simulink model "HW01_Tirel_Sim"  (R2020b)
settings: Solver=VariableStepAuto  StartTime=0.0  StopTime=1  RelTol=1e-3
values from neighbouring files (symbols this model uses):
  Bm = 1.02*10^-9    (= 1.02e-09)    [HW01_Tirel_Mat.m]
  Jm = 9.5*10^-10    (= 9.5e-10)    [HW01_Tirel_Mat.m]
  ke = 0.000114    [HW01_Tirel_Mat.m]
  km = 0.00109    [HW01_Tirel_Mat.m]
  La = 28*10^-6    (= 2.8e-05)    [HW01_Tirel_Mat.m]
  Ra = 8.8    [HW01_Tirel_Mat.m]
  Tl = ST/2    (= 0.000366)    [HW01_Tirel_Mat.m]
  Ts = 0.000011    (= 1.1e-05)    [HW01_Tirel_Mat.m]
undefined symbols (not defined in the file or in its folder): K, K1
libraries: simulink x4, cstblocks x2, pid_lib x2
settings Model: Creator=DELL  LastModifiedBy=DELL

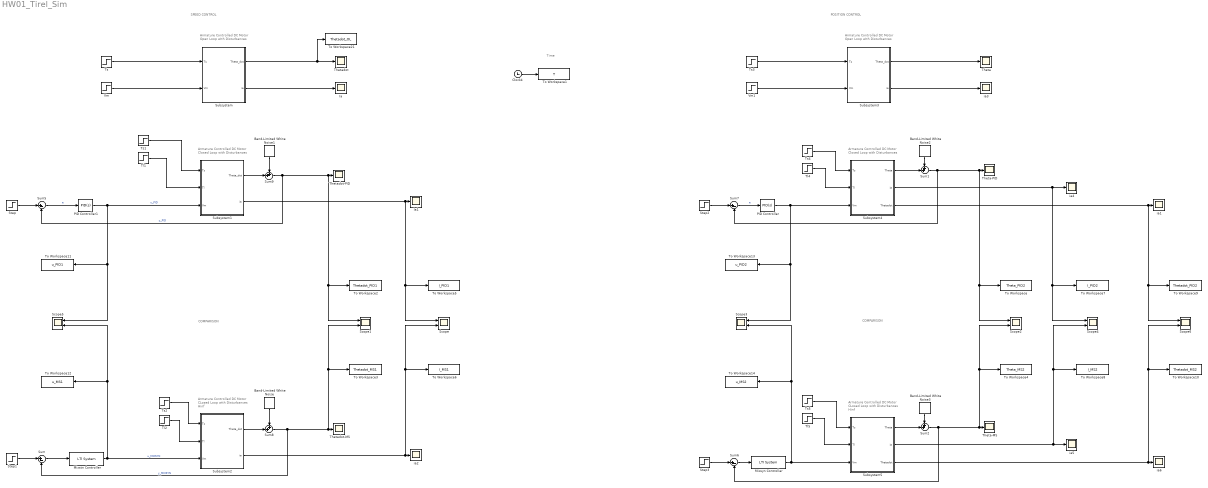
== system HW01_Tirel_Sim ==
  note: Time
  note: POSITION CONTROL
  note: SPEED CONTROL
  note: COMPARISON
  note: COMPARISON
  note: Armature Controlled DC Motor
      | Open Loop with Disturbances
  note: Armature Controlled DC Motor
      | Closed Loop with Disturbances
  note: Armature Controlled DC Motor
      | CLosed Loop with Disturbances Hinf
  note: Armature Controlled DC Motor
      | Open Loop with Disturbances
  note: Armature Controlled DC Motor
      | Closed Loop with Disturbances
  note: Armature Controlled DC Motor
      | CLosed Loop with Disturbances Hinf
  Band-Limited White Noise : simulink/Sources/Band-Limited White Noise  Cov=[0.001]  Ts=0.001  seed=[23341]
  Band-Limited White Noise1 : simulink/Sources/Band-Limited White Noise  Cov=[0.001]  Ts=0.001  seed=[23341]
  Band-Limited White Noise2 : simulink/Sources/Band-Limited White Noise  Cov=[0.00001]  Ts=0.001  seed=[23341]
  Band-Limited White Noise3 : simulink/Sources/Band-Limited White Noise  Cov=[0.00001]  Ts=0.001  seed=[23341]
  Clock4 : Clock
  Ia : Scope
  Ia1 : Scope
  Mixstn Controller : cstblocks/LTI System  sys=tf(K)  IC=[]
  Mixsyn Controller : cstblocks/LTI System  sys=tf(K1)  IC=[]
  PID Controller : pid_lib/PID Controller  Controller=PID  Form=Parallel  TimeDomain=Continuous-time  UseExternalTs=off  SampleTime=-1  IntegratorMethod=Forward Euler  FilterMethod=Forward Euler  ControllerParametersSource=internal  P=0.0298126781166158  I=0.262778070420961  D=0.000764301039173846  UseFilter=on  N=227.623795440392  TunerSelectOption=Transfer Function Based (PID Tuner App)  InitialConditionSource=internal  InitialConditionForIntegrator=0  InitialConditionForFilter=0  DifferentiatorICPrevScaledInput=0  ExternalReset=none  TrackingMode=off  Kt=1  LimitOutput=off  SatLimitsSource=internal  UpperSaturationLimit=inf  LowerSaturationLimit=-inf  LinearizeAsGain=on  AntiWindupMode=none  Kb=1  POutMin=[]  POutMax=[]  IOutMin=[]  IOutMax=[]  DOutMin=[]  DOutMax=[]  NOutMin=[]  NOutMax=[]  SumOutMin=[]  SumOutMax=[]  SaturationOutMin=[]  SaturationOutMax=[]  PParamMin=[]  PParamMax=[]  IParamMin=[]  IParamMax=[]  DParamMin=[]  DParamMax=[]  NParamMin=[]  NParamMax=[]  KbParamMin=[]  KbParamMax=[]  KtParamMin=[]  KtParamMax=[]  KbOutMin=[]  KbOutMax=[]  KtOutMin=[]  KtOutMax=[]  IntegratorOutMin=[]  IntegratorOutMax=[]  FilterOutMin=[]  FilterOutMax=[]  SumI1OutMin=[]  SumI1OutMax=[]  SumI2OutMin=[]  SumI2OutMax=[]  SumI3OutMin=[]  SumI3OutMax=[]  SumI4OutMin=[]  SumI4OutMax=[]  SumDOutMin=[]  SumDOutMax=[]  DifferentiatorOutMin=[]  DifferentiatorOutMax=[]  FilterDiffOutCoefMin=[]  FilterDiffOutCoefMax=[]  ReciprocalOutMin=[]  ReciprocalOutMax=[]  SumDenOutMin=[]  SumDenOutMax=[]  SumNumOutMin=[]  SumNumOutMax=[]  DivideOutMin=[]  DivideOutMax=[]  UdiffTsProdOutMin=[]  UdiffTsProdOutMax=[]  NTsProdOutMin=[]  NTsProdOutMax=[]  UintegralTsProdOutMin=[]  UintegralTsProdOutMax=[]  UngainTsProdOutMin=[]  UngainTsProdOutMax=[]  IntegratorContinuousStateAttributes=''  IntegratorStateMustResolveToSignalObject=off  IntegratorRTWStateStorageClass=Auto  FilterContinuousStateAttributes=''  FilterStateMustResolveToSignalObject=off  FilterRTWStateStorageClass=Auto  ParallelPVariant=InternalParameters  IdealPVariant=Disabled  IVariant=InternalParameters  DVariant=InternalParameters  IntegratorVariant=Continuous  SatVariant=Disabled  AWVariant=Passthrough  PCopyVariant=Disabled  TRVariant=Disabled  FdbkBlocksVariant=Forward  IdealPFdbkVariant=Disabled  SatFdbkVariant=Disabled  DerivativeFilterVariant=ContFilter  NVariant=InternalParameters  NCopyVariant=Disabled  FilterICVariant=InternalICsFilter  IntegratorICVariant=InternalICs  ExternalResetVariant=Disabled  TRSumVariant=Passthrough  SumFdbkVariant=Disabled  SumVariant=Sum_PID  TsampFilterVariant=InternalTs  TsampNgainVariant=Passthrough  TsampIntegralVariant=Passthrough  ExternalSaturationOutDataTypeStr=Inherit: Same as second input
  PID Controller1 : pid_lib/PID Controller  Controller=PID  Form=Parallel  TimeDomain=Continuous-time  UseExternalTs=off  SampleTime=-1  IntegratorMethod=Forward Euler  FilterMethod=Forward Euler  ControllerParametersSource=internal  P=0.000202128528554514  I=0.00612071081256607  D=-8.69937250601148e-07  UseFilter=on  N=32.3806372068654  TunerSelectOption=Transfer Function Based (PID Tuner App)  InitialConditionSource=internal  InitialConditionForIntegrator=0  InitialConditionForFilter=0  DifferentiatorICPrevScaledInput=0  ExternalReset=none  TrackingMode=off  Kt=1  LimitOutput=off  SatLimitsSource=internal  UpperSaturationLimit=inf  LowerSaturationLimit=-inf  LinearizeAsGain=on  AntiWindupMode=none  Kb=1  POutMin=[]  POutMax=[]  IOutMin=[]  IOutMax=[]  DOutMin=[]  DOutMax=[]  NOutMin=[]  NOutMax=[]  SumOutMin=[]  SumOutMax=[]  SaturationOutMin=[]  SaturationOutMax=[]  PParamMin=[]  PParamMax=[]  IParamMin=[]  IParamMax=[]  DParamMin=[]  DParamMax=[]  NParamMin=[]  NParamMax=[]  KbParamMin=[]  KbParamMax=[]  KtParamMin=[]  KtParamMax=[]  KbOutMin=[]  KbOutMax=[]  KtOutMin=[]  KtOutMax=[]  IntegratorOutMin=[]  IntegratorOutMax=[]  FilterOutMin=[]  FilterOutMax=[]  SumI1OutMin=[]  SumI1OutMax=[]  SumI2OutMin=[]  SumI2OutMax=[]  SumI3OutMin=[]  SumI3OutMax=[]  SumI4OutMin=[]  SumI4OutMax=[]  SumDOutMin=[]  SumDOutMax=[]  DifferentiatorOutMin=[]  DifferentiatorOutMax=[]  FilterDiffOutCoefMin=[]  FilterDiffOutCoefMax=[]  ReciprocalOutMin=[]  ReciprocalOutMax=[]  SumDenOutMin=[]  SumDenOutMax=[]  SumNumOutMin=[]  SumNumOutMax=[]  DivideOutMin=[]  DivideOutMax=[]  UdiffTsProdOutMin=[]  UdiffTsProdOutMax=[]  NTsProdOutMin=[]  NTsProdOutMax=[]  UintegralTsProdOutMin=[]  UintegralTsProdOutMax=[]  UngainTsProdOutMin=[]  UngainTsProdOutMax=[]  IntegratorContinuousStateAttributes=''  IntegratorStateMustResolveToSignalObject=off  IntegratorRTWStateStorageClass=Auto  FilterContinuousStateAttributes=''  FilterStateMustResolveToSignalObject=off  FilterRTWStateStorageClass=Auto  ParallelPVariant=InternalParameters  IdealPVariant=Disabled  IVariant=InternalParameters  DVariant=InternalParameters  IntegratorVariant=Continuous  SatVariant=Disabled  AWVariant=Passthrough  PCopyVariant=Disabled  TRVariant=Disabled  FdbkBlocksVariant=Forward  IdealPFdbkVariant=Disabled  SatFdbkVariant=Disabled  DerivativeFilterVariant=ContFilter  NVariant=InternalParameters  NCopyVariant=Disabled  FilterICVariant=InternalICsFilter  IntegratorICVariant=InternalICs  ExternalResetVariant=Disabled  TRSumVariant=Passthrough  SumFdbkVariant=Disabled  SumVariant=Sum_PID  TsampFilterVariant=InternalTs  TsampNgainVariant=Passthrough  TsampIntegralVariant=Passthrough  ExternalSaturationOutDataTypeStr=Inherit: Same as second input
  Scope{,1..6} (7 alike) : Scope  NumInputPorts=2
  Step : Step  Time=0  After=25000  SampleTime=0
  Step1 : Step  Time=0  After=25000  SampleTime=0
  Step2 : Step  Time=0  After=210  SampleTime=0
  Step3 : Step  Time=0  After=210  SampleTime=0
  Subsystem : Subsystem
  Subsystem1 : Subsystem
  Subsystem2 : Subsystem
  Subsystem3 : Subsystem
  Subsystem4 : Subsystem
  Subsystem5 : Subsystem
  Sum{,5..7} (4 alike) : Sum  Inputs=|+-
  Sum{1..2,8..9} (4 alike) : Sum  Inputs=++|
  Theta : Scope
  Theta-MS : Scope
  Theta-PID : Scope
  Thetadot : Scope
  Thetadot-MS : Scope
  Thetadot-PID : Scope
  Tl{1..2,4..5} (4 alike) : Step  Time=0.5  After=Tl  SampleTime=0
  To Workspace : ToWorkspace  VariableName=Theta_PID2  SampleTime=-1
  To Workspace1 : ToWorkspace  VariableName=T  SampleTime=-1
  To Workspace10 : ToWorkspace  VariableName=Thetadot_MS2  SampleTime=-1
  To Workspace11 : ToWorkspace  VariableName=u_PID1  SampleTime=-1
  To Workspace12 : ToWorkspace  VariableName=u_MS1  SampleTime=-1
  To Workspace13 : ToWorkspace  VariableName=u_PID2  SampleTime=-1
  To Workspace14 : ToWorkspace  VariableName=u_MS2  SampleTime=-1
  To Workspace2 : ToWorkspace  VariableName=Thetadot_PID1  SampleTime=-1
  To Workspace21 : ToWorkspace  VariableName=Thetadot_OL  SampleTime=-1
  To Workspace3 : ToWorkspace  VariableName=Thetadot_MS1  SampleTime=-1
  To Workspace4 : ToWorkspace  VariableName=Theta_MS2  SampleTime=-1
  To Workspace5 : ToWorkspace  VariableName=I_PID1  SampleTime=-1
  To Workspace6 : ToWorkspace  VariableName=I_MS1  SampleTime=-1
  To Workspace7 : ToWorkspace  VariableName=I_PID2  SampleTime=-1
  To Workspace8 : ToWorkspace  VariableName=I_MS2  SampleTime=-1
  To Workspace9 : ToWorkspace  VariableName=Thetadot_PID2  SampleTime=-1
  Ts{,1..5} (6 alike) : Step  Time=0  After=Ts  SampleTime=0
  Vm : Step  Time=0  After=6  SampleTime=0
  Vm1 : Step  Time=0  After=6  SampleTime=0
  ia{1..6} (6 alike) : Scope
  wires:
  Vm/1 -> Subsystem/2(Vm)
  Subsystem/1(Theta_dot) -> To Workspace21/1, Thetadot/1
  Subsystem/2(ia) -> Ia/1
  Ts1/1 -> Subsystem1/1(Ts)
  Subsystem1/2(ia) -> Scope/1, To Workspace5/1, Ia1/1
  Sum5/1 -> PID Controller1/1  "e"
  PID Controller1/1 -> Scope5/1, To Workspace11/1, Subsystem1/3(Vm)  "u_PID"
  Subsystem2/2(ia) -> To Workspace6/1, Scope/2, ia2/1
  Ts2/1 -> Subsystem2/1(Ts)
  Tl2/1 -> Subsystem2/2(Tl)
  Mixstn Controller/1 -> Subsystem2/3(Vm), To Workspace12/1, Scope5/2  "u_MIXSYN"
  Sum/1 -> Mixstn Controller/1
  Sum6/1 -> Mixsyn Controller/1
  Tl5/1 -> Subsystem5/2(Tl)
  Ts5/1 -> Subsystem5/1(Ts)
  Subsystem5/2(ia) -> ia5/1, To Workspace8/1, Scope4/2
  Sum7/1 -> PID Controller/1  "e"
  Tl4/1 -> Subsystem4/2(Tl)
  Subsystem3/2(ia) -> ia3/1
  Ts4/1 -> Subsystem4/1(Ts)
  Mixsyn Controller/1 -> Subsystem5/3(Vm), To Workspace14/1, Scope3/2
  Vm1/1 -> Subsystem3/2(Vm)
  Subsystem3/1(Theta_dot) -> Theta/1
  Ts/1 -> Subsystem/1(Ts)
  Tl1/1 -> Subsystem1/2(Tl)
  Ts3/1 -> Subsystem3/1(Ts)
  Step1/1 -> Sum/1
  Step/1 -> Sum5/1
  Sum8/1 -> Sum/2, To Workspace3/1, Scope1/2, Thetadot-MS/1  "y_MIXSYN"
  Sum9/1 -> Sum5/2, Scope1/1, To Workspace2/1, Thetadot-PID/1  "y_PID"
  PID Controller/1 -> To Workspace13/1, Scope3/1, Subsystem4/3(Vm)
  Sum2/1 -> Sum6/2, To Workspace4/1, Scope2/2, Theta-MS/1
  Step3/1 -> Sum6/1
  Step2/1 -> Sum7/1
  Clock4/1 -> To Workspace1/1
  Subsystem4/2(ia) -> To Workspace7/1, Scope4/1, ia4/1
  Subsystem1/1(Theta_dot) -> Sum9/2
  Band-Limited White Noise1/1 -> Sum9/1
  Subsystem2/1(Theta_dot) -> Sum8/2
  Band-Limited White Noise/1 -> Sum8/1
  Subsystem5/1(Theta) -> Sum2/2
  Subsystem5/3(Thetadot) -> Scope6/2, To Workspace10/1, ia6/1
  Subsystem4/3(Thetadot) -> To Workspace9/1, Scope6/1, ia1/1
  Subsystem4/1(Theta) -> Sum1/2
  Sum1/1 -> Sum7/2, To Workspace/1, Scope2/1, Theta-PID/1
  Band-Limited White Noise2/1 -> Sum1/1
  Band-Limited White Noise3/1 -> Sum2/1

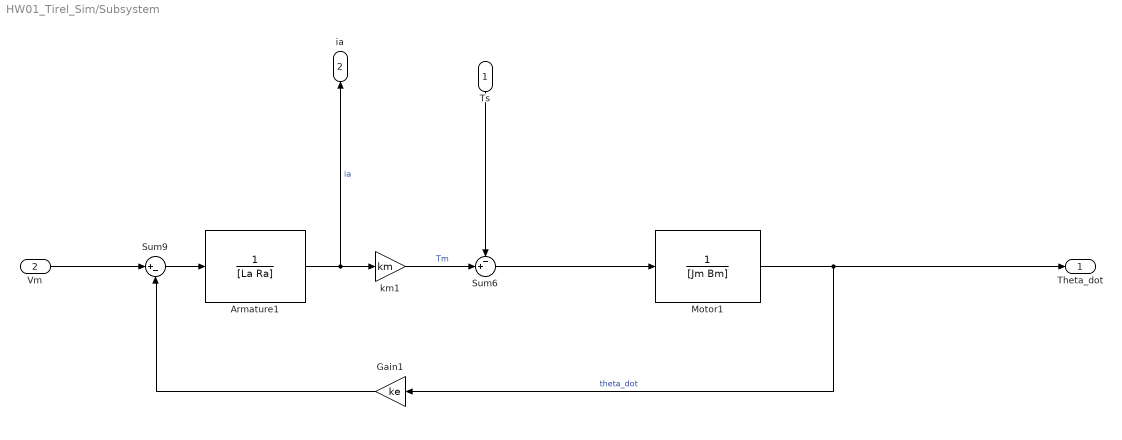
== system HW01_Tirel_Sim/Subsystem ==
  Ts : Inport
  Vm : Inport  Port=2
  Armature1 : TransferFcn  Denominator=[La Ra]
  Gain1 : Gain  Gain=ke
  Motor1 : TransferFcn  Denominator=[Jm Bm]
  Sum6 : Sum  Inputs=-+|
  Sum9 : Sum  Inputs=|+-
  km1 : Gain  Gain=km
  Theta_dot : Outport
  ia : Outport  Port=2
  wires:
  Sum9/1 -> Armature1/1
  Gain1/1 -> Sum9/2
  Armature1/1 -> ia/1, km1/1  "ia"
  Motor1/1 -> Theta_dot/1, Gain1/1  "theta_dot"
  Sum6/1 -> Motor1/1
  km1/1 -> Sum6/2  "Tm"
  Vm/1 -> Sum9/1
  Ts/1 -> Sum6/1

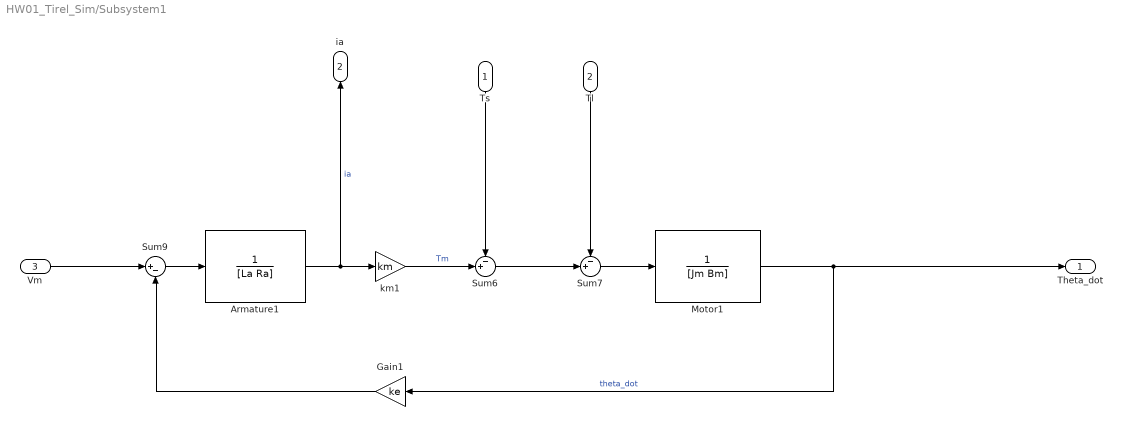
== system HW01_Tirel_Sim/Subsystem1 ==
  Ts : Inport
  Tl : Inport  Port=2
  Vm : Inport  Port=3
  Armature1 : TransferFcn  Denominator=[La Ra]
  Gain1 : Gain  Gain=ke
  Motor1 : TransferFcn  Denominator=[Jm Bm]
  Sum6 : Sum  Inputs=-+|
  Sum7 : Sum  Inputs=-+|
  Sum9 : Sum  Inputs=|+-
  km1 : Gain  Gain=km
  Theta_dot : Outport
  ia : Outport  Port=2
  wires:
  Sum9/1 -> Armature1/1
  Gain1/1 -> Sum9/2
  Armature1/1 -> ia/1, km1/1  "ia"
  Motor1/1 -> Theta_dot/1, Gain1/1  "theta_dot"
  Sum6/1 -> Sum7/2
  Sum7/1 -> Motor1/1
  Tl/1 -> Sum7/1
  km1/1 -> Sum6/2  "Tm"
  Vm/1 -> Sum9/1
  Ts/1 -> Sum6/1

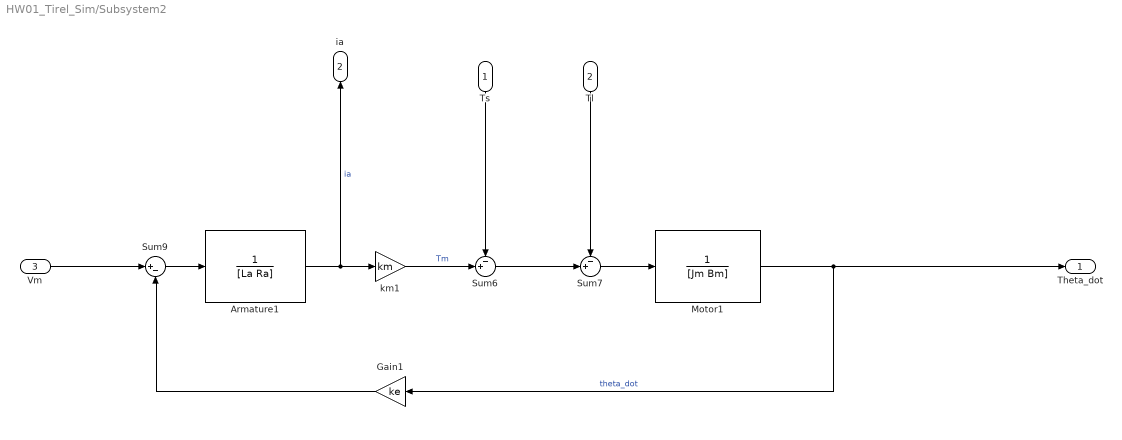
== system HW01_Tirel_Sim/Subsystem2 ==
  Ts : Inport
  Tl : Inport  Port=2
  Vm : Inport  Port=3
  Armature1 : TransferFcn  Denominator=[La Ra]
  Gain1 : Gain  Gain=ke
  Motor1 : TransferFcn  Denominator=[Jm Bm]
  Sum6 : Sum  Inputs=-+|
  Sum7 : Sum  Inputs=-+|
  Sum9 : Sum  Inputs=|+-
  km1 : Gain  Gain=km
  Theta_dot : Outport
  ia : Outport  Port=2
  wires:
  Sum9/1 -> Armature1/1
  Gain1/1 -> Sum9/2
  Armature1/1 -> ia/1, km1/1  "ia"
  Motor1/1 -> Theta_dot/1, Gain1/1  "theta_dot"
  Sum6/1 -> Sum7/2
  Sum7/1 -> Motor1/1
  Tl/1 -> Sum7/1
  km1/1 -> Sum6/2  "Tm"
  Vm/1 -> Sum9/1
  Ts/1 -> Sum6/1

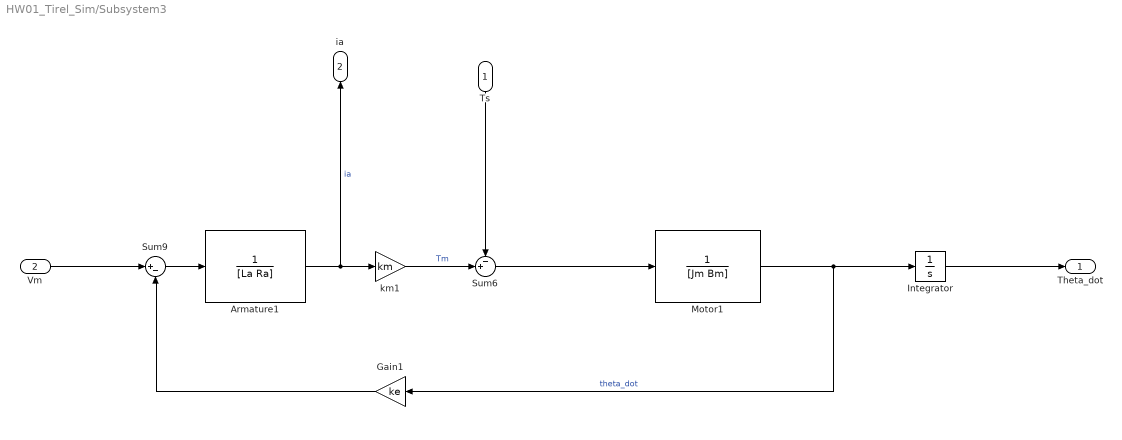
== system HW01_Tirel_Sim/Subsystem3 ==
  Ts : Inport
  Vm : Inport  Port=2
  Armature1 : TransferFcn  Denominator=[La Ra]
  Gain1 : Gain  Gain=ke
  Integrator : Integrator
  Motor1 : TransferFcn  Denominator=[Jm Bm]
  Sum6 : Sum  Inputs=-+|
  Sum9 : Sum  Inputs=|+-
  km1 : Gain  Gain=km
  Theta_dot : Outport
  ia : Outport  Port=2
  wires:
  Sum9/1 -> Armature1/1
  Gain1/1 -> Sum9/2
  Armature1/1 -> ia/1, km1/1  "ia"
  Motor1/1 -> Integrator/1, Gain1/1  "theta_dot"
  Sum6/1 -> Motor1/1
  km1/1 -> Sum6/2  "Tm"
  Vm/1 -> Sum9/1
  Ts/1 -> Sum6/1
  Integrator/1 -> Theta_dot/1

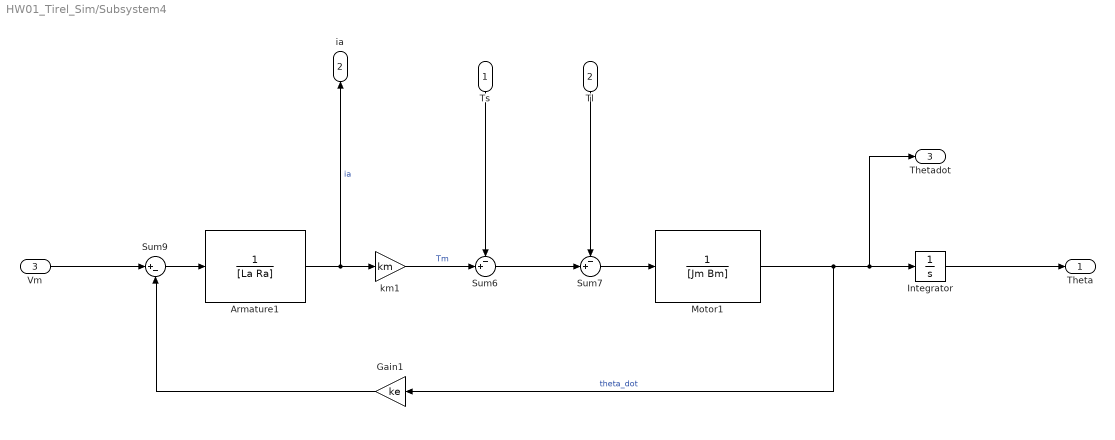
== system HW01_Tirel_Sim/Subsystem4 ==
  Ts : Inport
  Tl : Inport  Port=2
  Vm : Inport  Port=3
  Armature1 : TransferFcn  Denominator=[La Ra]
  Gain1 : Gain  Gain=ke
  Integrator : Integrator
  Motor1 : TransferFcn  Denominator=[Jm Bm]
  Sum6 : Sum  Inputs=-+|
  Sum7 : Sum  Inputs=-+|
  Sum9 : Sum  Inputs=|+-
  km1 : Gain  Gain=km
  Theta : Outport
  ia : Outport  Port=2
  Thetadot : Outport  Port=3
  wires:
  Sum9/1 -> Armature1/1
  Gain1/1 -> Sum9/2
  Armature1/1 -> ia/1, km1/1  "ia"
  Motor1/1 -> Integrator/1, Thetadot/1, Gain1/1  "theta_dot"
  Sum6/1 -> Sum7/2
  Sum7/1 -> Motor1/1
  Tl/1 -> Sum7/1
  km1/1 -> Sum6/2  "Tm"
  Vm/1 -> Sum9/1
  Ts/1 -> Sum6/1
  Integrator/1 -> Theta/1

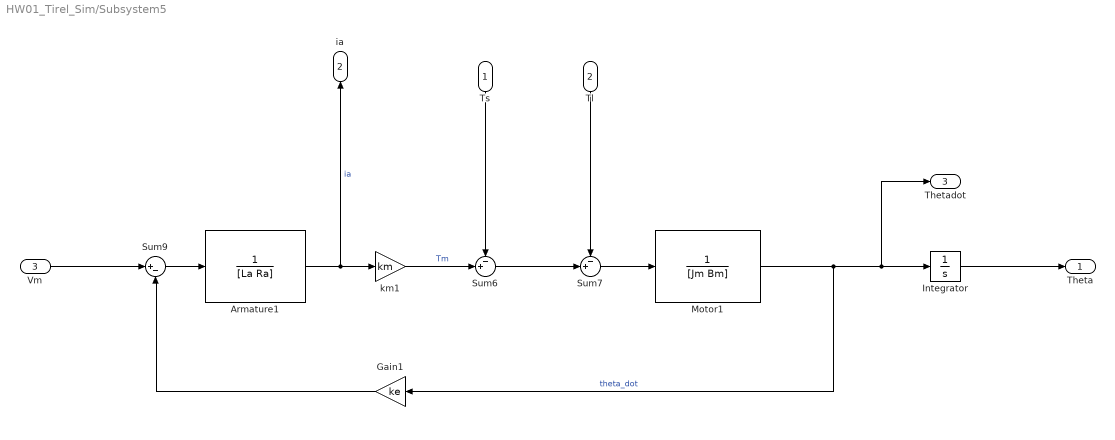
== system HW01_Tirel_Sim/Subsystem5 ==
  Ts : Inport
  Tl : Inport  Port=2
  Vm : Inport  Port=3
  Armature1 : TransferFcn  Denominator=[La Ra]
  Gain1 : Gain  Gain=ke
  Integrator : Integrator
  Motor1 : TransferFcn  Denominator=[Jm Bm]
  Sum6 : Sum  Inputs=-+|
  Sum7 : Sum  Inputs=-+|
  Sum9 : Sum  Inputs=|+-
  km1 : Gain  Gain=km
  Theta : Outport
  ia : Outport  Port=2
  Thetadot : Outport  Port=3
  wires:
  Sum9/1 -> Armature1/1
  Gain1/1 -> Sum9/2
  Armature1/1 -> ia/1, km1/1  "ia"
  Motor1/1 -> Integrator/1, Thetadot/1, Gain1/1  "theta_dot"
  Sum6/1 -> Sum7/2
  Sum7/1 -> Motor1/1
  Tl/1 -> Sum7/1
  km1/1 -> Sum6/2  "Tm"
  Vm/1 -> Sum9/1
  Ts/1 -> Sum6/1
  Integrator/1 -> Theta/1
